simulink model "Work2WithTraffic"  (R2015b)
settings: Solver=FixedStepDiscrete  StartTime=0.0  StopTime=300  FixedStep=1  RelTol=1e-3
settings Model: Creator=Irina_Novokhatskay  LastModifiedBy=Druzhinin_Vasily

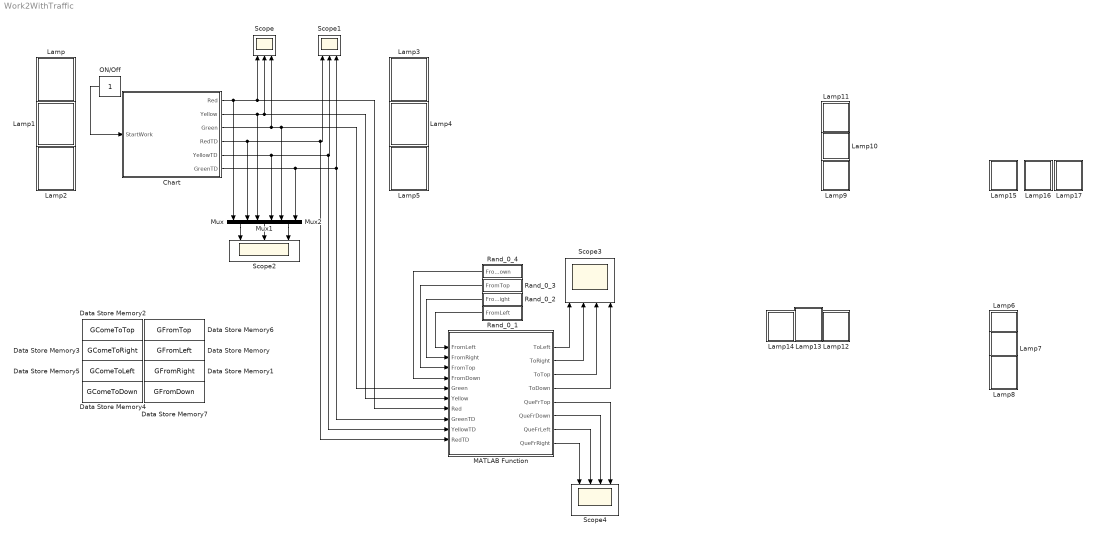
== system Work2WithTraffic ==
  Chart : Stateflow chart  TreatAsAtomicUnit=on  mask{LRTimeGreen=20, TDTimeGreen=20}
  Data Store Memory : DataStoreMemory  DataStoreName=GFromLeft  ReadBeforeWriteMsg=warning  WriteAfterWriteMsg=warning  WriteAfterReadMsg=warning  OutDataTypeStr=double
  Data Store Memory1 : DataStoreMemory  DataStoreName=GFromRight  ReadBeforeWriteMsg=warning  WriteAfterWriteMsg=warning  WriteAfterReadMsg=warning  OutDataTypeStr=double
  Data Store Memory2 : DataStoreMemory  DataStoreName=GComeToTop  ReadBeforeWriteMsg=warning  WriteAfterWriteMsg=warning  WriteAfterReadMsg=warning  OutDataTypeStr=double
  Data Store Memory3 : DataStoreMemory  DataStoreName=GComeToRight  ReadBeforeWriteMsg=warning  WriteAfterWriteMsg=warning  WriteAfterReadMsg=warning  OutDataTypeStr=double
  Data Store Memory4 : DataStoreMemory  DataStoreName=GComeToDown  ReadBeforeWriteMsg=warning  WriteAfterWriteMsg=warning  WriteAfterReadMsg=warning  OutDataTypeStr=double
  Data Store Memory5 : DataStoreMemory  DataStoreName=GComeToLeft  ReadBeforeWriteMsg=warning  WriteAfterWriteMsg=warning  WriteAfterReadMsg=warning  OutDataTypeStr=double
  Data Store Memory6 : DataStoreMemory  DataStoreName=GFromTop  ReadBeforeWriteMsg=warning  WriteAfterWriteMsg=warning  WriteAfterReadMsg=warning  OutDataTypeStr=double
  Data Store Memory7 : DataStoreMemory  DataStoreName=GFromDown  ReadBeforeWriteMsg=warning  WriteAfterWriteMsg=warning  WriteAfterReadMsg=warning  OutDataTypeStr=double
  Lamp : Subsystem  DialogController=hmiCreateDDGDialog  IsWebBlock=on  mask(MWDashboardBlock){webBlockId=6a72cd25-3ace-4f89-9e8c-9b6b07c39fc1, webBlockType=lamp, ShowInLibBrowser=on, ShowInitialText=on, HMISrcModelName=Work2WithTraffic}
      mask prompts: webBlockType "WebBlock Type"; HMISrcModelName "Source Model"
      mask Help: helpview([docroot '/mapfiles/simulink.map'], 'hmi_lamp')
      mask Display:
      | if strcmp(get_param(bdroot(gcb),'BlockDiagramType'), 'library')
      |     image([(matlabroot) '/toolbox/simulink/hmi/icons/Lamp.png']);
      | end
  Lamp1 : Subsystem  DialogController=hmiCreateDDGDialog  IsWebBlock=on  mask(MWDashboardBlock){webBlockId=0b83c74a-5baa-4a76-abe6-b8eaac528e0c, webBlockType=lamp, ShowInLibBrowser=on, ShowInitialText=on, HMISrcModelName=Work2WithTraffic}
      mask prompts: webBlockType "WebBlock Type"; HMISrcModelName "Source Model"
      mask Help: helpview([docroot '/mapfiles/simulink.map'], 'hmi_lamp')
      mask Display:
      | if strcmp(get_param(bdroot(gcb),'BlockDiagramType'), 'library')
      |     image([(matlabroot) '/toolbox/simulink/hmi/icons/Lamp.png']);
      | end
  Lamp10 : Subsystem  DialogController=hmiCreateDDGDialog  IsWebBlock=on  mask(MWDashboardBlock){webBlockId=15f45251-5f67-42fd-ba7a-edb8e11b9a6a, webBlockType=lamp, ShowInLibBrowser=on, ShowInitialText=on, HMISrcModelName=Work2WithTraffic}
      mask prompts: webBlockType "WebBlock Type"; HMISrcModelName "Source Model"
      mask Help: helpview([docroot '/mapfiles/simulink.map'], 'hmi_lamp')
      mask Display:
      | if strcmp(get_param(bdroot(gcb),'BlockDiagramType'), 'library')
      |     image([(matlabroot) '/toolbox/simulink/hmi/icons/Lamp.png']);
      | end
  Lamp11 : Subsystem  DialogController=hmiCreateDDGDialog  IsWebBlock=on  mask(MWDashboardBlock){webBlockId=2de18072-848c-4ef7-bacd-9321842b3b74, webBlockType=lamp, ShowInLibBrowser=on, ShowInitialText=on, HMISrcModelName=Work2WithTraffic}
      mask prompts: webBlockType "WebBlock Type"; HMISrcModelName "Source Model"
      mask Help: helpview([docroot '/mapfiles/simulink.map'], 'hmi_lamp')
      mask Display:
      | if strcmp(get_param(bdroot(gcb),'BlockDiagramType'), 'library')
      |     image([(matlabroot) '/toolbox/simulink/hmi/icons/Lamp.png']);
      | end
  Lamp12 : Subsystem  DialogController=hmiCreateDDGDialog  IsWebBlock=on  mask(MWDashboardBlock){webBlockId=f8163705-30c2-478c-bfca-d909051ab481, webBlockType=lamp, ShowInLibBrowser=on, ShowInitialText=on, HMISrcModelName=Work2WithTraffic}
      mask prompts: webBlockType "WebBlock Type"; HMISrcModelName "Source Model"
      mask Help: helpview([docroot '/mapfiles/simulink.map'], 'hmi_lamp')
      mask Display:
      | if strcmp(get_param(bdroot(gcb),'BlockDiagramType'), 'library')
      |     image([(matlabroot) '/toolbox/simulink/hmi/icons/Lamp.png']);
      | end
  Lamp13 : Subsystem  DialogController=hmiCreateDDGDialog  IsWebBlock=on  mask(MWDashboardBlock){webBlockId=fc402684-b095-4abc-a5ce-f123ecd30ffe, webBlockType=lamp, ShowInLibBrowser=on, ShowInitialText=on, HMISrcModelName=Work2WithTraffic}
      mask prompts: webBlockType "WebBlock Type"; HMISrcModelName "Source Model"
      mask Help: helpview([docroot '/mapfiles/simulink.map'], 'hmi_lamp')
      mask Display:
      | if strcmp(get_param(bdroot(gcb),'BlockDiagramType'), 'library')
      |     image([(matlabroot) '/toolbox/simulink/hmi/icons/Lamp.png']);
      | end
  Lamp14 : Subsystem  DialogController=hmiCreateDDGDialog  IsWebBlock=on  mask(MWDashboardBlock){webBlockId=a8644dce-0fa4-41a3-b5a3-b7ded4881562, webBlockType=lamp, ShowInLibBrowser=on, ShowInitialText=on, HMISrcModelName=Work2WithTraffic}
      mask prompts: webBlockType "WebBlock Type"; HMISrcModelName "Source Model"
      mask Help: helpview([docroot '/mapfiles/simulink.map'], 'hmi_lamp')
      mask Display:
      | if strcmp(get_param(bdroot(gcb),'BlockDiagramType'), 'library')
      |     image([(matlabroot) '/toolbox/simulink/hmi/icons/Lamp.png']);
      | end
  Lamp15 : Subsystem  DialogController=hmiCreateDDGDialog  IsWebBlock=on  mask(MWDashboardBlock){webBlockId=7805cf90-d16b-4850-aef1-ca00daf5dcb3, webBlockType=lamp, ShowInLibBrowser=on, ShowInitialText=on, HMISrcModelName=Work2WithTraffic}
      mask prompts: webBlockType "WebBlock Type"; HMISrcModelName "Source Model"
      mask Help: helpview([docroot '/mapfiles/simulink.map'], 'hmi_lamp')
      mask Display:
      | if strcmp(get_param(bdroot(gcb),'BlockDiagramType'), 'library')
      |     image([(matlabroot) '/toolbox/simulink/hmi/icons/Lamp.png']);
      | end
  Lamp16 : Subsystem  DialogController=hmiCreateDDGDialog  IsWebBlock=on  mask(MWDashboardBlock){webBlockId=0230a9b6-90f6-42b8-9fba-191a9e515e07, webBlockType=lamp, ShowInLibBrowser=on, ShowInitialText=on, HMISrcModelName=Work2WithTraffic}
      mask prompts: webBlockType "WebBlock Type"; HMISrcModelName "Source Model"
      mask Help: helpview([docroot '/mapfiles/simulink.map'], 'hmi_lamp')
      mask Display:
      | if strcmp(get_param(bdroot(gcb),'BlockDiagramType'), 'library')
      |     image([(matlabroot) '/toolbox/simulink/hmi/icons/Lamp.png']);
      | end
  Lamp17 : Subsystem  DialogController=hmiCreateDDGDialog  IsWebBlock=on  mask(MWDashboardBlock){webBlockId=8a785a16-254f-44fb-8cfe-09d7cf8042f9, webBlockType=lamp, ShowInLibBrowser=on, ShowInitialText=on, HMISrcModelName=Work2WithTraffic}
      mask prompts: webBlockType "WebBlock Type"; HMISrcModelName "Source Model"
      mask Help: helpview([docroot '/mapfiles/simulink.map'], 'hmi_lamp')
      mask Display:
      | if strcmp(get_param(bdroot(gcb),'BlockDiagramType'), 'library')
      |     image([(matlabroot) '/toolbox/simulink/hmi/icons/Lamp.png']);
      | end
  Lamp2 : Subsystem  DialogController=hmiCreateDDGDialog  IsWebBlock=on  mask(MWDashboardBlock){webBlockId=e27a65a0-1e4d-4ed1-96a1-defa4afd1051, webBlockType=lamp, ShowInLibBrowser=on, ShowInitialText=on, HMISrcModelName=Work2WithTraffic}
      mask prompts: webBlockType "WebBlock Type"; HMISrcModelName "Source Model"
      mask Help: helpview([docroot '/mapfiles/simulink.map'], 'hmi_lamp')
      mask Display:
      | if strcmp(get_param(bdroot(gcb),'BlockDiagramType'), 'library')
      |     image([(matlabroot) '/toolbox/simulink/hmi/icons/Lamp.png']);
      | end
  Lamp3 : Subsystem  DialogController=hmiCreateDDGDialog  IsWebBlock=on  mask(MWDashboardBlock){webBlockId=9a19c506-71ae-4a57-994f-6279ef339d96, webBlockType=lamp, ShowInLibBrowser=on, ShowInitialText=on, HMISrcModelName=Work2WithTraffic}
      mask prompts: webBlockType "WebBlock Type"; HMISrcModelName "Source Model"
      mask Help: helpview([docroot '/mapfiles/simulink.map'], 'hmi_lamp')
      mask Display:
      | if strcmp(get_param(bdroot(gcb),'BlockDiagramType'), 'library')
      |     image([(matlabroot) '/toolbox/simulink/hmi/icons/Lamp.png']);
      | end
  Lamp4 : Subsystem  DialogController=hmiCreateDDGDialog  IsWebBlock=on  mask(MWDashboardBlock){webBlockId=34e4b4fc-f0f9-4732-bebf-acbc3324067c, webBlockType=lamp, ShowInLibBrowser=on, ShowInitialText=on, HMISrcModelName=Work2WithTraffic}
      mask prompts: webBlockType "WebBlock Type"; HMISrcModelName "Source Model"
      mask Help: helpview([docroot '/mapfiles/simulink.map'], 'hmi_lamp')
      mask Display:
      | if strcmp(get_param(bdroot(gcb),'BlockDiagramType'), 'library')
      |     image([(matlabroot) '/toolbox/simulink/hmi/icons/Lamp.png']);
      | end
  Lamp5 : Subsystem  DialogController=hmiCreateDDGDialog  IsWebBlock=on  mask(MWDashboardBlock){webBlockId=46939de4-5fc6-4d9b-a5f7-006a554046a3, webBlockType=lamp, ShowInLibBrowser=on, ShowInitialText=on, HMISrcModelName=Work2WithTraffic}
      mask prompts: webBlockType "WebBlock Type"; HMISrcModelName "Source Model"
      mask Help: helpview([docroot '/mapfiles/simulink.map'], 'hmi_lamp')
      mask Display:
      | if strcmp(get_param(bdroot(gcb),'BlockDiagramType'), 'library')
      |     image([(matlabroot) '/toolbox/simulink/hmi/icons/Lamp.png']);
      | end
  Lamp6 : Subsystem  DialogController=hmiCreateDDGDialog  IsWebBlock=on  mask(MWDashboardBlock){webBlockId=41663ddb-bc88-46f9-83ac-f1e7484bb24e, webBlockType=lamp, ShowInLibBrowser=on, ShowInitialText=on, HMISrcModelName=Work2WithTraffic}
      mask prompts: webBlockType "WebBlock Type"; HMISrcModelName "Source Model"
      mask Help: helpview([docroot '/mapfiles/simulink.map'], 'hmi_lamp')
      mask Display:
      | if strcmp(get_param(bdroot(gcb),'BlockDiagramType'), 'library')
      |     image([(matlabroot) '/toolbox/simulink/hmi/icons/Lamp.png']);
      | end
  Lamp7 : Subsystem  DialogController=hmiCreateDDGDialog  IsWebBlock=on  mask(MWDashboardBlock){webBlockId=3a8707aa-c691-48fb-b5ca-e343ac96153c, webBlockType=lamp, ShowInLibBrowser=on, ShowInitialText=on, HMISrcModelName=Work2WithTraffic}
      mask prompts: webBlockType "WebBlock Type"; HMISrcModelName "Source Model"
      mask Help: helpview([docroot '/mapfiles/simulink.map'], 'hmi_lamp')
      mask Display:
      | if strcmp(get_param(bdroot(gcb),'BlockDiagramType'), 'library')
      |     image([(matlabroot) '/toolbox/simulink/hmi/icons/Lamp.png']);
      | end
  Lamp8 : Subsystem  DialogController=hmiCreateDDGDialog  IsWebBlock=on  mask(MWDashboardBlock){webBlockId=01bae4a3-615c-4b87-9642-9742c6fff1f3, webBlockType=lamp, ShowInLibBrowser=on, ShowInitialText=on, HMISrcModelName=Work2WithTraffic}
      mask prompts: webBlockType "WebBlock Type"; HMISrcModelName "Source Model"
      mask Help: helpview([docroot '/mapfiles/simulink.map'], 'hmi_lamp')
      mask Display:
      | if strcmp(get_param(bdroot(gcb),'BlockDiagramType'), 'library')
      |     image([(matlabroot) '/toolbox/simulink/hmi/icons/Lamp.png']);
      | end
  Lamp9 : Subsystem  DialogController=hmiCreateDDGDialog  IsWebBlock=on  mask(MWDashboardBlock){webBlockId=79ace46e-a0a5-4d52-b8a3-0b07a0b6810c, webBlockType=lamp, ShowInLibBrowser=on, ShowInitialText=on, HMISrcModelName=Work2WithTraffic}
      mask prompts: webBlockType "WebBlock Type"; HMISrcModelName "Source Model"
      mask Help: helpview([docroot '/mapfiles/simulink.map'], 'hmi_lamp')
      mask Display:
      | if strcmp(get_param(bdroot(gcb),'BlockDiagramType'), 'library')
      |     image([(matlabroot) '/toolbox/simulink/hmi/icons/Lamp.png']);
      | end
  MATLAB Function : MATLAB Function  TreatAsAtomicUnit=on
  Mux : Mux  Inputs=2
  Mux1 : Mux  Inputs=2
  Mux2 : Mux  Inputs=2
  ON/Off : Constant  OutDataTypeStr=boolean
  Rand_0_1 : Subsystem  mask{Par=3}
  Rand_0_2 : Subsystem  mask{Par=3}
  Rand_0_3 : Subsystem  mask{Par=3}
  Rand_0_4 : Subsystem  mask{Par=3}
  Scope : Scope  NumInputPorts=3
  Scope1 : Scope  NumInputPorts=3
  Scope2 : Scope  NumInputPorts=3
  Scope3 : Scope  NumInputPorts=4
  Scope4 : Scope  NumInputPorts=4
  wires:
  Chart/1(Red) -> MATLAB Function/7(Red), Scope/1, Mux/1
  Chart/2(Yellow) -> MATLAB Function/6(Yellow), Scope/2, Mux1/1
  Chart/3(Green) -> Scope/3, MATLAB Function/5(Green), Mux2/1
  Chart/4(RedTD) -> MATLAB Function/10(RedTD), Scope1/1, Mux/2
  Chart/5(YellowTD) -> MATLAB Function/9(YellowTD), Scope1/2, Mux1/2
  Chart/6(GreenTD) -> Scope1/3, MATLAB Function/8(GreenTD), Mux2/2
  Mux/1 -> Scope2/1
  Mux1/1 -> Scope2/2
  Mux2/1 -> Scope2/3
  ON/Off/1 -> Chart/1(StartWork)
  MATLAB Function/7(QueFrLeft) -> Scope4/2
  MATLAB Function/8(QueFrRight) -> Scope4/1
  MATLAB Function/1(ToLeft) -> Scope3/1
  MATLAB Function/2(ToRight) -> Scope3/2
  MATLAB Function/3(ToTop) -> Scope3/3
  MATLAB Function/4(ToDown) -> Scope3/4
  Rand_0_2/1(FromRight) -> MATLAB Function/2(FromRight)
  MATLAB Function/6(QueFrDown) -> Scope4/3
  MATLAB Function/5(QueFrTop) -> Scope4/4
  Rand_0_3/1(FromTop) -> MATLAB Function/3(FromTop)
  Rand_0_4/1(FromDown) -> MATLAB Function/4(FromDown)
  Rand_0_1/1(FromLeft) -> MATLAB Function/1(FromLeft)

== system Work2WithTraffic/Lamp ==

== system Work2WithTraffic/Lamp1 ==

== system Work2WithTraffic/Lamp10 ==

== system Work2WithTraffic/Lamp11 ==

== system Work2WithTraffic/Lamp12 ==

== system Work2WithTraffic/Lamp13 ==

== system Work2WithTraffic/Lamp14 ==

== system Work2WithTraffic/Lamp15 ==

== system Work2WithTraffic/Lamp16 ==

== system Work2WithTraffic/Lamp17 ==

== system Work2WithTraffic/Lamp2 ==

== system Work2WithTraffic/Lamp3 ==

== system Work2WithTraffic/Lamp4 ==

== system Work2WithTraffic/Lamp5 ==

== system Work2WithTraffic/Lamp6 ==

== system Work2WithTraffic/Lamp7 ==

== system Work2WithTraffic/Lamp8 ==

== system Work2WithTraffic/Lamp9 ==

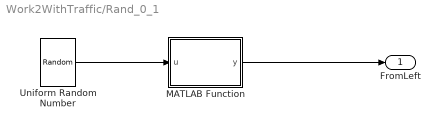
== system Work2WithTraffic/Rand_0_1 ==
  MATLAB Function : MATLAB Function  TreatAsAtomicUnit=on
  Uniform Random Number : UniformRandomNumber  Minimum=0  Maximum=Par  Seed=4  SampleTime=1
  FromLeft : Outport
  wires:
  Uniform Random Number/1 -> MATLAB Function/1(u)
  MATLAB Function/1(y) -> FromLeft/1

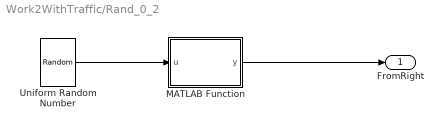
== system Work2WithTraffic/Rand_0_2 ==
  MATLAB Function : MATLAB Function  TreatAsAtomicUnit=on
  Uniform Random Number : UniformRandomNumber  Minimum=0  Maximum=Par  Seed=3  SampleTime=1
  FromRight : Outport
  wires:
  MATLAB Function/1(y) -> FromRight/1
  Uniform Random Number/1 -> MATLAB Function/1(u)

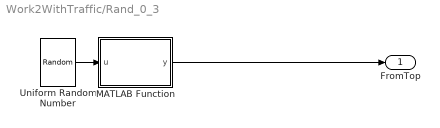
== system Work2WithTraffic/Rand_0_3 ==
  MATLAB Function : MATLAB Function  TreatAsAtomicUnit=on
  Uniform Random Number : UniformRandomNumber  Minimum=0  Maximum=Par  Seed=2  SampleTime=1
  FromTop : Outport
  wires:
  MATLAB Function/1(y) -> FromTop/1
  Uniform Random Number/1 -> MATLAB Function/1(u)

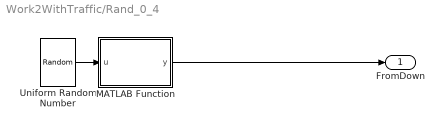
== system Work2WithTraffic/Rand_0_4 ==
  MATLAB Function : MATLAB Function  TreatAsAtomicUnit=on
  Uniform Random Number : UniformRandomNumber  Minimum=0  Maximum=Par  Seed=1  SampleTime=1
  FromDown : Outport
  wires:
  Uniform Random Number/1 -> MATLAB Function/1(u)
  MATLAB Function/1(y) -> FromDown/1

== matlab function Work2WithTraffic/MATLAB Function ==
  data: FromLeft input; FromRight input; FromTop input; FromDown input; ToLeft output; ToRight output; ToTop output; ToDown output; QueFrTop output; QueFrDown output; GFromLeft data_store_memory; Green input; Yellow input; Red input; GComeToTop data_store_memory; GComeToRight data_store_memory; GComeToDown data_store_memory; QueFrLeft output; GFromRight data_store_memory; GComeToLeft data_store_memory; QueFrRight output; GFromTop data_store_memory; GFromDown data_store_memory; GreenTD input; YellowTD input; RedTD input
function [ToLeft,ToRight,ToTop,ToDown,QueFrTop,QueFrDown, QueFrLeft,QueFrRight] = fcn(FromLeft,FromRight,FromTop,FromDown,Green,Yellow,Red,GreenTD,YellowTD,RedTD)
%#codegen
ParamToTurnLeft = 1;
ParamToGoFront = 2;
ParamToGoRight =1;

global GFromLeft;
global GFromRight;
global GFromTop;
global GFromDown;

global GComeToDown;
global GComeToTop;
global GComeToRight;
global GComeToLeft;


% From Top To Other ---------------------------------------------------
GFromTop = AddToQueue(GFromTop,FromTop);
[FromTopToRight,FromTopToDown,FromTopToLeft,GFromTop]=TraficLogic(RedTD,YellowTD,GreenTD,GFromTop,ParamToTurnLeft,ParamToGoFront,ParamToGoRight);  
%----------------------------------------------------------------------

%From left to other-----------------------------------------------------
GFromLeft = AddToQueue(GFromLeft,FromLeft);
[FromLeftToTop,FromLeftToRight,FromLeftToDown,GFromLeft]=TraficLogic(Red,Yellow,Green,GFromLeft,ParamToTurnLeft,ParamToGoFront,ParamToGoRight);  
%------------------------------------------------------------------------

% From Right To Other ---------------------------------------------------
GFromRight = AddToQueue(GFromRight,FromRight);
[FromRightToDown,FromRightToLeft,FromRightToTop,GFromRight]=TraficLogic(Red,Yellow,Green,GFromRight,ParamToTurnLeft,ParamToGoFront,ParamToGoRight);
%------------------------------------------------------------------------

% From Down To Other ---------------------------------------------------
GFromDown = AddToQueue(GFromDown,FromDown);
[FromDownToLeft,FromDownToTop,FromDownToRight,GFromDown]=TraficLogic(RedTD,YellowTD,GreenTD,GFromDown,ParamToTurnLeft,ParamToGoFront,ParamToGoRight);  
%----------------------------------------------------------------------


% Total Calc
QueFrLeft = GFromLeft;
QueFrRight = GFromRight;
QueFrTop = GFromTop;
QueFrDown = GFromDown;

GComeToTop = GComeToTop + FromLeftToTop + FromRightToTop + FromDownToTop;
ToTop = GComeToTop;
GComeToRight = GComeToRight + FromLeftToRight + FromTopToRight + FromDownToRight;
ToRight = GComeToRight;
GComeToDown = GComeToDown + FromLeftToDown + FromRightToDown + FromTopToDown;
ToDown= GComeToDown;
GComeToLeft = GComeToLeft + FromRightToLeft + FromTopToLeft + FromDownToLeft;
ToLeft = GComeToLeft;

== matlab function Work2WithTraffic/Rand_0_1/MATLAB Function ==
  data: u input; y output
function y = fcn(u)
%#codegen
y = ToInt(u);

== stateflow chart Work2WithTraffic/Chart ==
  state Controler
    state TrafickLiteLogic [parallel]
      settings: executionOrder=1
      state YellowBlink1
        entry: Red=0;
        Yellow=0;
        Green=0;
      state YellowBlink
        entry: Red=0;
        Yellow=1;
        Green=0;
      state Red
        entry: Red=1;
        Yellow = 0;
        Green=0;
        state RedAndYellow
          entry:
          Red =1;
          Yellow=1;
          Green = 0;
          Block=true;
        state Delay
          entry:
          Turn=false;
        (default) -> Delay
        Delay -> RedAndYellow : [Turn]
      state Yellow
        entry:
        Red=0;
        Yellow=1;
        Green=0;
      state GreenBlink1
        entry:
        Red=0;
        Yellow=0;
        Green=0;
        GBL = GBL + 1;
      state GreenBlink
        entry:
        Red=0;
        Yellow=0;
        Green=1;
      state Green
        entry:
        Red=0;
        Yellow=0;
        Green=1;
        GBL = 0;
      (default) -> YellowBlink
      YellowBlink -> YellowBlink1 [order 1] : [after(1,sec) && ~StartWork]
      YellowBlink1 -> YellowBlink : after(1,sec)
      YellowBlink -> RedAndYellow [order 2] : [StartWork]
      RedAndYellow -> Green : after(LRTimeGreen,sec)
      Yellow -> Red : after(5,sec)
      GreenBlink -> Yellow [order 2] : [GBL==3]
      GreenBlink -> GreenBlink1 [order 1] : [after(1,sec) &&GBL~=3 ]
      GreenBlink1 -> GreenBlink : after(1,sec)
      Green -> GreenBlink : after(40,sec)
    state TrafickLiteLogic1 [parallel]
      settings: executionOrder=2
      state YellowBlink1TD
        entry: RedTD=0;
        YellowTD=0;
        GreenTD=0;
      state YellowBlinkTD
        entry: RedTD=0;
        YellowTD=1;
        GreenTD=0;
      state RedTD
        entry: RedTD=1;
        YellowTD = 0;
        GreenTD=0;
        state RedAndYellowTD
          entry:
          RedTD =1;
          YellowTD=1;
          GreenTD = 0;
          Block=true;
        state DelayTD
          entry:
          Turn=true;
        DelayTD -> RedAndYellowTD : [~Turn]
        (default) -> DelayTD
      state YellowTD
        entry:
        RedTD=0;
        YellowTD=1;
        GreenTD=0;
      state GreenBlink1TD
        entry:
        RedTD=0;
        YellowTD=0;
        GreenTD=0;
        GBLTD = GBLTD + 1;
      state GreenBlinkTD
        entry:
        RedTD=0;
        YellowTD=0;
        GreenTD=1;
      state GreenTD
        entry:
        RedTD=0;
        YellowTD=0;
        GreenTD=1;
        GBLTD = 0;
      (default) -> YellowBlinkTD
      YellowBlinkTD -> YellowBlink1TD [order 1] : [after(1,sec) && ~StartWork]
      YellowBlink1TD -> YellowBlinkTD : after(1,sec)
      YellowBlinkTD -> RedTD [order 2] : [StartWork]
      RedAndYellowTD -> GreenTD : after(TDTimeGreen,sec)
      YellowTD -> RedTD : after(5,sec)
      GreenBlinkTD -> YellowTD [order 2] : [GBLTD==3]
      GreenBlinkTD -> GreenBlink1TD [order 1] : [after(1,sec) &&GBLTD~=3 ]
      GreenBlink1TD -> GreenBlinkTD : after(1,sec)
      GreenTD -> GreenBlinkTD : after(40,sec)
  data: Red output; Yellow output; Green output; GBL local; RedTD output; YellowTD output; GreenTD output; GBLTD local; Turn local boolean; StartWork input boolean; Block local boolean; LRTimeGreen parameter; TDTimeGreen parameter

== matlab function Work2WithTraffic/Rand_0_2/MATLAB Function ==
  data: u input; y output
function y = fcn(u)
%#codegen
y = ToInt(u);

== matlab function Work2WithTraffic/Rand_0_3/MATLAB Function ==
  data: u input; y output
function y = fcn(u)
%#codegen
y = ToInt(u);

== matlab function Work2WithTraffic/Rand_0_4/MATLAB Function ==
  data: u input; y output
function y = fcn(u)
%#codegen
y = ToInt(u);
